simulink model "FK_Arman"  (R2020a)
settings: Solver=FixedStepDiscrete  StartTime=0.0  StopTime=500  FixedStep=0.1  RelTol=1e-3
StopFcn:
  | aero_radplot_dsp;
model workspace (MAT data in the model file):
  deltat = 1
  g = 32.2
  speed = 700
  tauT = 4
  tauc = 5
undefined symbols (not defined in the file or in its folder): DiscIntNeverNeededParam
libraries: simulink x2, dspadpt3 x1
CloseFcn:
  | radarFigureHandles=findall(0,'type','figure','tag','aero_radplot_dsp');if ~isempty(radarFigureHandles);close(radarFigureHandles);end
  | clear radarFigureHandles;
  | if exist('radarLogsOut');clear radarLogsOut;end;
settings Model: OrderedModelArguments=off  Creator=arman  LastModifiedBy=arman
settings DataIOCC: SaveFormat=Array  SaveOutput=off  SaveTime=off  ReturnWorkspaceOutputs=off  TimeSaveName=t_sim  SignalLoggingName=radarLogsOut
settings SFSimCC: CustomCodeUndefinedFunction=UseInterfaceOnly

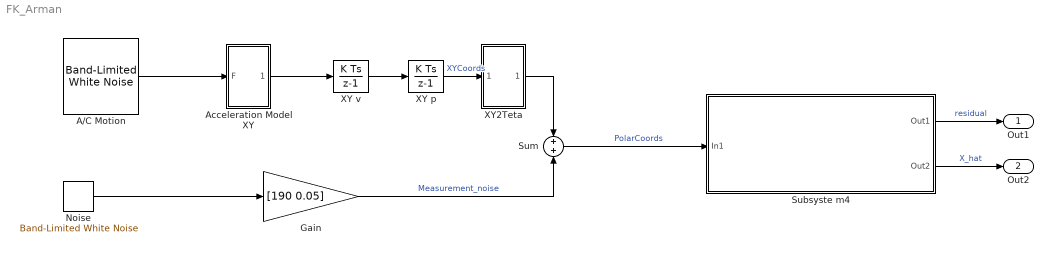
== system FK_Arman ==
  A/C Motion : simulink/Sources/Band-Limited White Noise  Cov=[0 0]  Ts=0.1  seed=[0 0]  mask(Band-Limited White Noise.){}
      mask Display: image('D:\airplane.png'); % Use "Edit Image" on toolstrip to change.
  Acceleration Model XY : Subsystem
  Gain : Gain  Gain=[190 0.05]
  Noise : simulink/Sources/Band-Limited White Noise  Cov=[1 1]  Ts=0.1  seed=[1 1]
  Subsyste m4 : Subsystem
  Sum : Sum  OutDataTypeStr=Inherit: Same as first input
  XY p : DiscreteIntegrator  InitialCondition=[0, speed]  SampleTime=-1  ICPrevOutput=DiscIntNeverNeededParam  ICPrevScaledInput=DiscIntNeverNeededParam
  XY v : DiscreteIntegrator  InitialCondition=[0, speed]  SampleTime=-1  ICPrevOutput=DiscIntNeverNeededParam  ICPrevScaledInput=DiscIntNeverNeededParam
  XY2Teta : Subsystem
  Out1 : Outport  VectorParamsAs1DForOutWhenUnconnected=off
  Out2 : Outport  Port=2  VectorParamsAs1DForOutWhenUnconnected=off
  wires:
  A/C Motion/1 -> Acceleration Model XY/1(F)
  Acceleration Model XY/1(Out1) -> XY v/1
  XY v/1 -> XY p/1
  XY p/1 -> XY2Teta/1(XY1)  "XYCoords"
  Noise/1 -> Gain/1
  Gain/1 -> Sum/2  "Measurement_noise"
  Sum/1 -> Subsyste m4/1(In1)  "PolarCoords"
  Subsyste m4/2(Out2) -> Out2/1  "X_hat"
  Subsyste m4/1(Out1) -> Out1/1  "residual"
  XY2Teta/1(Out1) -> Sum/1

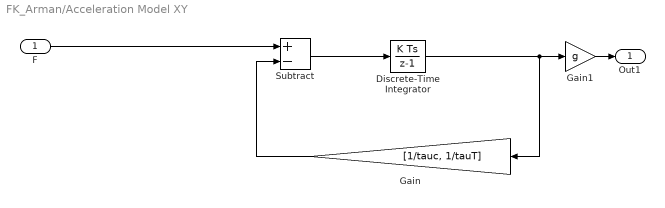
== system FK_Arman/Acceleration Model XY ==
  F : Inport
  Discrete-Time Integrator : DiscreteIntegrator  SampleTime=-1  ICPrevOutput=DiscIntNeverNeededParam  ICPrevScaledInput=DiscIntNeverNeededParam
  Gain : Gain  Gain=[1/tauc, 1/tauT]
  Gain1 : Gain  Gain=g
  Subtract : Sum  Inputs=+-
  Out1 : Outport  VectorParamsAs1DForOutWhenUnconnected=off
  wires:
  Discrete-Time Integrator/1 -> Gain/1, Gain1/1
  Gain1/1 -> Out1/1
  Gain/1 -> Subtract/2
  Subtract/1 -> Discrete-Time Integrator/1
  F/1 -> Subtract/1

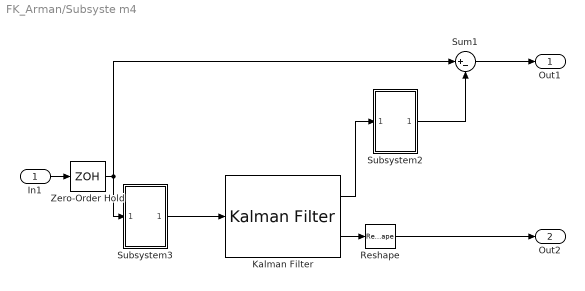
== system FK_Arman/Subsyste m4 ==
  In1 : Inport
  Kalman Filter : dspadpt3/Kalman Filter  num_targets=1  sourceEnable=Always  isReset=on  X=[0.001; 0.01; 0.001; 400]  P=zeros(4)  A=[1 deltat 0 0; 0 1 0 0 ; 0 0 1 deltat; 0 0 0 1]  sourceMeasure=Specify via Dialog  H=[1 0 0 0; 0 0 1 0]  Q=diag([0 0.005 0 0.005])  R=300*eye(2)  isOutputEstMeasure=on  isOutputEstState=on  isOutputEstError=off  isOutputPrdMeasure=off  isOutputPrdState=off  isOutputPrdError=off
      settings: SourceProductBaseCode=DS
  Reshape : Reshape
  Subsystem2 : Subsystem
  Subsystem3 : Subsystem
  Sum1 : Sum  Inputs=|+-
  Zero-Order Hold : ZeroOrderHold  SampleTime=deltat
  Out1 : Outport  VectorParamsAs1DForOutWhenUnconnected=off
  Out2 : Outport  Port=2  VectorParamsAs1DForOutWhenUnconnected=off
  wires:
  Zero-Order Hold/1 -> Subsystem3/1(In1), Sum1/1
  Sum1/1 -> Out1/1
  In1/1 -> Zero-Order Hold/1
  Subsystem2/1(Out1) -> Sum1/2
  Kalman Filter/2 -> Reshape/1
  Kalman Filter/1 -> Subsystem2/1(XY1)
  Reshape/1 -> Out2/1
  Subsystem3/1(Out1) -> Kalman Filter/1

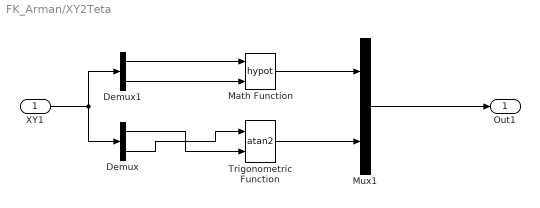
== system FK_Arman/XY2Teta ==
  XY1 : Inport
  Demux : Demux  Outputs=2
  Demux1 : Demux  Outputs=2
  Math Function : Math  Operator=hypot  SignedPower=on  OutputSignalType=real  SaturateOnIntegerOverflow=on
  Mux1 : Mux  Inputs=2
  Trigonometric Function : Trigonometry  Operator=atan2  OutputSignalType=real
  Out1 : Outport  PortDimensions=2  VectorParamsAs1DForOutWhenUnconnected=off
  wires:
  Demux/1 -> Trigonometric Function/2
  Demux/2 -> Trigonometric Function/1
  Demux1/1 -> Math Function/1
  Demux1/2 -> Math Function/2
  XY1/1 -> Demux/1, Demux1/1
  Mux1/1 -> Out1/1
  Math Function/1 -> Mux1/1
  Trigonometric Function/1 -> Mux1/2

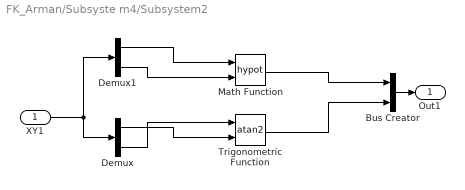
== system FK_Arman/Subsyste m4/Subsystem2 ==
  XY1 : Inport
  Bus Creator : BusCreator  Inputs=2
  Demux : Demux  Outputs=2
  Demux1 : Demux  Outputs=2
  Math Function : Math  Operator=hypot  SignedPower=on  SaturateOnIntegerOverflow=on
  Trigonometric Function : Trigonometry  Operator=atan2
  Out1 : Outport  VectorParamsAs1DForOutWhenUnconnected=off
  wires:
  Math Function/1 -> Bus Creator/1
  Demux/1 -> Trigonometric Function/2
  Demux/2 -> Trigonometric Function/1
  Demux1/1 -> Math Function/1
  Bus Creator/1 -> Out1/1
  Demux1/2 -> Math Function/2
  Trigonometric Function/1 -> Bus Creator/2
  XY1/1 -> Demux/1, Demux1/1

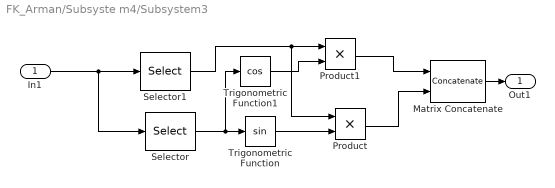
== system FK_Arman/Subsyste m4/Subsystem3 ==
  In1 : Inport
  Matrix Concatenate : Concatenate  ConcatenateDimension=2
  Product : Product
  Product1 : Product
  Selector : Selector  InputPortWidth=2  IndexOptions=Index vector (dialog)  Indices=[2]  OutputSizes=1
  Selector1 : Selector  InputPortWidth=2  IndexOptions=Index vector (dialog)  Indices=[1]  OutputSizes=1
  Trigonometric Function : Trigonometry
  Trigonometric Function1 : Trigonometry  Operator=cos
  Out1 : Outport  VectorParamsAs1DForOutWhenUnconnected=off
  wires:
  Matrix Concatenate/1 -> Out1/1
  Selector1/1 -> Product/1, Product1/1
  In1/1 -> Selector1/1, Selector/1
  Selector/1 -> Trigonometric Function/1, Trigonometric Function1/1
  Product/1 -> Matrix Concatenate/2
  Trigonometric Function1/1 -> Product1/2
  Product1/1 -> Matrix Concatenate/1
  Trigonometric Function/1 -> Product/2
